simulink model "untitled"  (R2017b)
settings: Solver=FixedStepAuto  StartTime=0.0  StopTime=0.08  FixedStep=5e-6  RelTol=1e-3
undefined symbols (not defined in the file): fdesignblkfcn, gcbh
libraries: simulink x1, dspfdesign x1, dsparch4 x1, powerlib x1
(part 2 of 3)

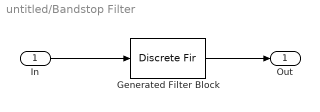
== system untitled/Bandstop Filter ==
  In : Inport
  Generated Filter Block : DiscreteFir  Tag=BlockMethodSubSystem  Coefficients=[0.0223633707576158421 -0.00133514714885774629 -0.00129522874823918637 -0.00125157131765571829 -0.0012111989449531328 -0.00116715419445947554 -0.00112656054179939721 -0.00108232798172859372 -0.00104173239829644148 -0.000997513459988745447 -0.000957132044750909003 -0.000913097287102123192 -0.000873138256319086264 -0.000829449599907571868 -0.000790117727737720682 -0.000746907127080915882 -0.000708402771521067748 -0.000665799144441112621 -0.000628318718468144134 -0.000586411493907609371 -0.000550162121436673091 -0.000509014189946773712 -0.000474217796990226016 -0.000433817926332199231 -0.000400763524282300189 -0.000360999851043220085 -0.000330100833889800528 -0.000290611199089457837 -0.000262651271772653024 -0.000222321795588145915 -0.000199455971541505253 -0.000151749452218149741 -0.000143683642153048563 -0.000120753831814615276 -4.72713574370204812e-05 -3.80794804504107308e-05 -1.10668539518232324e-05 3.04222394216286294e-06 3.03703838969967238e-05 5.10152243656154881e-05 7.95941368107720454e-05 0.000102259009395945418 0.000129227984267990369 0.000150568992412993864 0.000174235772647565897 0.000192903162671418212 0.000213012463608534158 0.000228980720148371186 0.000246051806526522332 0.000259869183754456395 0.000274630070705523133 0.000286882966519790006 0.000299909100629818773 0.000311005114267793193 0.000322614086292717585 0.000332708538205959536 0.000342962415560100044 0.000352050924203263309 0.000360829002791505753 0.000368825371198959571 0.000375880430830911514 0.000382787615328930705 0.000387691629451338558 0.000394079806824541997 0.00039357994666734138 0.000406576275282830349 0.000401378881451668035 0.000398504108523616951 0.000405453723465673446 0.000406234549465405359 0.000407408752059109974 0.000403495216011361439 0.000401073670190933566 0.000396175307062426722 0.000393494008388892266 0.000389041673356605843 0.000386289642012677343 0.000381513479089235614 0.000377756028105504936 0.000371796133781546905 0.000366587318726335992 0.000359330357465712728 0.000352895805747345461 0.000344742222520246953 0.00033758675706264897 0.000328978514045189126 0.000321459915361103064 0.000312605465883870632 0.000304832989400561586 0.000295679158065368384 0.000287560882449745781 0.000277934092341900916 0.00026935919034650678 0.000259076927852891264 0.000250043284540820896 0.00023890892073610907 0.000229663960957948726 0.000218859638669800165 0.000204780455879150999 0.000199197888731641337 0.000186362360106910141 0.000173571260309902454 0.00016183758324915339 0.000151530227221580507 0.00014141327808027442 0.000130806741710893327 0.000119775667598283713 0.000108292200612421558 9.7080658579903786e-05 8.59673054330868614e-05 7.55301186427180494e-05 6.51878818380484225e-05 5.53744799466703738e-05 4.53430957006656566e-05 3.56537928439423465e-05 2.55817200596600854e-05 1.58876450258033713e-05 5.87502897087770436e-06 -3.54736834108660186e-06 -1.31558544866307346e-05 -2.19837377175329214e-05 -3.09544278301496123e-05 -3.90271981338644695e-05 -4.73488416117729701e-05 -5.46979714893629018e-05 -6.25249808592591975e-05 -6.91918498269073948e-05 -7.67601131476653266e-05 -8.24853622630840398e-05 -9.05331341084707566e-05 -9.48870945500316103e-05 -0.000101129418356141383 -0.000108946069125713491 -0.000112326586618339904 -0.000117089758790750939 -0.000121722103591991076 -0.000127120624541717593 -0.000131248590481443053 -0.000135041096802513105 -0.000137873130958127995 -0.000140874382971071176 -0.000143559688651363933 -0.000146528929029977233 -0.000149093743435843259 -0.000151595292671997804 -0.000153457075964279509 -0.000155095291418468761 -0.000156156325999332198 -0.000157083179991499488 -0.000157601655756138597 -0.000158066072793411653 -0.000158183667495919052 -0.000158184593632602183 -0.000157769267389132496 -0.000157140161725435971 -0.000156040807638285463 -0.000154686467075110565 -0.000152897680659257401 -0.000150901092474636344 -0.000148595086767154398 -0.000146099605950373901 -0.00014366133298807256 -0.000140065505892049424 -0.00013881015253248467 ...(+48250 chars)]  InputProcessing=Columns as channels (frame based)
  Out : Outport
  wires:
  Generated Filter Block/1 -> Out/1
  In/1 -> Generated Filter Block/1
